simulink model "sensor"  (R2016b)
settings: Solver=FixedStepDiscrete  StartTime=0.0  StopTime=10.0  RelTol=1e-3
undefined symbols (not defined in the file): ObservationNoise, SpeedOfLight
settings Model: Creator=csax  LastModifiedBy=csax
settings OptimizationCC: DefaultParameterBehavior=Inlined
settings DebuggingCC: ParameterTunabilityLossMsg=error
settings HardwareCC: ProdBitPerPointer=32  ProdBitPerSizeT=32  ProdBitPerPtrDiffT=32  ProdLargestAtomicFloat=None  ProdWordSize=32  ProdHWDeviceType=Custom Processor->Custom
settings RTWCC: SystemTargetFile=trace32_target_ert.tlc  MakeCommand=trace32_target_make  TemplateMakefile=trace32_arm_tmf.tmf  Description=TRACE32 Target  GenerateReport=on  IncludeHyperlinkInReport=on  LaunchReport=on  GenerateTraceInfo=on  GenerateTraceReport=on  GenerateTraceReportSl=on  GenerateTraceReportSf=on  GenerateTraceReportEml=on
settings CodeAppCC: ForceParamTrailComments=on  IgnoreCustomStorageClasses=off  OperatorAnnotations=on  SimulinkDataObjDesc=on  SFDataObjDesc=on  MATLABFcnDesc=on  InsertBlockDesc=on  MATLABSourceComments=on
settings STFCustomTargetCC: TargetLangStandard=C99 (ISO)  CombineOutputUpdateFcns=on  ERTCustomFileBanners=on  SupportContinuousTime=off  SupportNonInlinedSFcns=off  RemoveResetFunc=on  MATLABClassNameForMDSCustomization=Simulink.SoftwareTarget.ERTCustomization  GRTInterface=off  SystemTargetFile=trace32_target_ert.tlc
settings ERTTargetCC: TargetLangStandard=C99 (ISO)  ParMdlRefBuildCompliant=off  CompOptLevelCompliant=off  ConcurrentExecutionCompliant=off  ERTFirstTimeCompliant=off  ModelStepFunctionPrototypeControlCompliant=off  CPPClassGenCompliant=off  UseToolchainInfoCompliant=off  InlinedParameterPlacement=NonHierarchical  ERTCustomFileTemplate=example_file_process.tlc

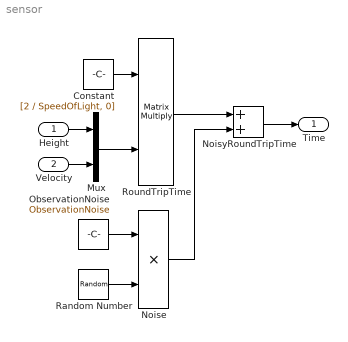
== system sensor ==
  Height : Inport
  Velocity : Inport  Port=2
  Constant : Constant  Value=[2 / SpeedOfLight, 0]  VectorParams1D=off  SampleTime=-1
  Mux : Mux  Inputs=2
  Noise : Product
  NoisyRoundTripTime : Sum
  ObservationNoise : Constant  Value=ObservationNoise
  Random Number : RandomNumber  SampleTime=0.1
  RoundTripTime : Product  Multiplication=Matrix(*)
  Time : Outport
  wires:
  Height/1 -> Mux/1
  Velocity/1 -> Mux/2
  Mux/1 -> RoundTripTime/2
  Constant/1 -> RoundTripTime/1
  ObservationNoise/1 -> Noise/1
  Random Number/1 -> Noise/2
  Noise/1 -> NoisyRoundTripTime/2
  RoundTripTime/1 -> NoisyRoundTripTime/1
  NoisyRoundTripTime/1 -> Time/1
